simulink model "powers"  (Simulink 5.0)
settings: Solver=ode45  SolverMode=SingleTasking  StartTime=0.0  StopTime=0.2  RelTol=1e-4  AbsTol=1e-8
CloseFcn:
  | ;slview('closediagram',bdroot);
settings Model: LastModifiedBy=Blue Phoenix  LimitDataPoints=off  BlockReductionOpt=off  BooleanDataType=off

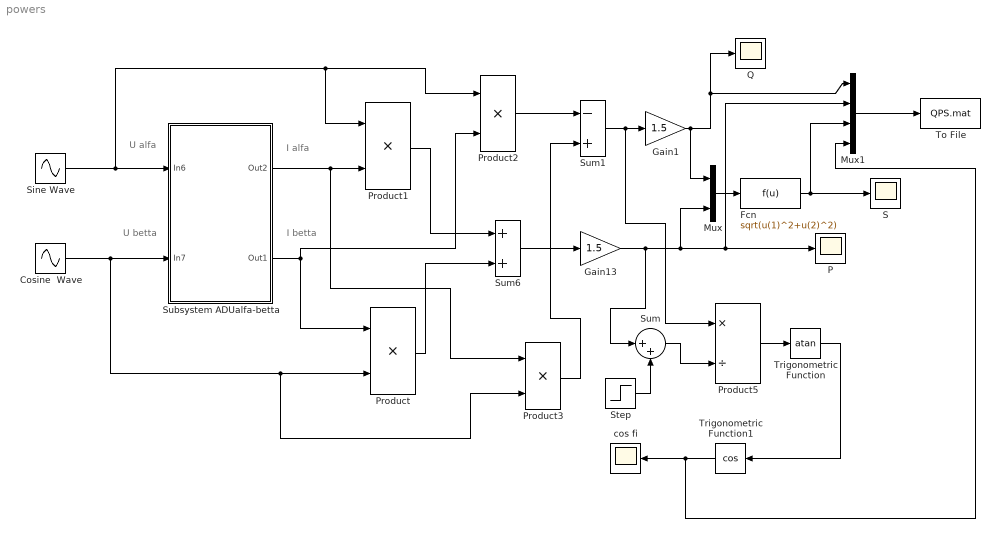
== system powers ==
  note: I alfa
  note: I betta
  note: U alfa
  note: U betta
  "  Q" : Scope
      settings: TickLabels=on  TimeRange=80  YMin=-1  YMax=2  SaveName=ScopeData3  DataFormat=Array
  "  S" : Scope
      settings: TickLabels=on  TimeRange=80  YMin=-1  YMax=2  SaveName=ScopeData5  DataFormat=Array
  " P" : Scope
      settings: TickLabels=on  TimeRange=80  YMin=-1  YMax=2  SaveName=ScopeData2  DataFormat=Array
  Cosine  Wave : Sin  Amplitude=311  Frequency=314  Phase=-pi/2  SampleTime=0
  Fcn : Fcn  Expr=sqrt(u(1)^2+u(2)^2)
  Gain1 : Gain  Gain=1.5  SaturateOnIntegerOverflow=on
  Gain13 : Gain  Gain=1.5  SaturateOnIntegerOverflow=on
  Mux : Mux  Inputs=2
  Mux1 : Mux
  Product{,1..3} (4 alike) : Product  SaturateOnIntegerOverflow=on  InputSameDT=on
  Product5 : Product  Inputs=*/  SaturateOnIntegerOverflow=on  InputSameDT=on
  Sine Wave : Sin  Amplitude=311  Frequency=314  SampleTime=0
  Step : Step  Time=0.001  Before=0.0001  After=0  SampleTime=0
  Subsystem ADUalfa-betta : Subsystem
  Sum : Sum  Inputs=|++  SaturateOnIntegerOverflow=on  InputSameDT=on
  Sum1 : Sum  Inputs=-+  SaturateOnIntegerOverflow=on  InputSameDT=on
  Sum6 : Sum  SaturateOnIntegerOverflow=on  InputSameDT=on
  To File : ToFile  Filename=QPS.mat
  Trigonometric Function : Trigonometry  Operator=atan
  Trigonometric Function1 : Trigonometry  Orientation=left  Operator=cos
  cos fi : Scope
      settings: TickLabels=on  TimeRange=0.1  YMin=-1  YMax=2  SaveName=ScopeData4  DataFormat=Array
  wires:
  Subsystem ADUalfa-betta/1(Out2) -> Product1/2, Product3/1
  Sine Wave/1 -> Subsystem ADUalfa-betta/1(In6), Product1/1, Product2/1
  Cosine  Wave/1 -> Subsystem ADUalfa-betta/2(In7), Product/2, Product3/2
  Subsystem ADUalfa-betta/2(Out1) -> Product/1, Product2/2
  Product1/1 -> Sum6/1
  Product/1 -> Sum6/2
  Gain13/1 -> Sum/1, Mux/2, " P"/1, Mux1/2
  Sum6/1 -> Gain13/1
  Product3/1 -> Sum1/2
  Product2/1 -> Sum1/1
  Sum1/1 -> Gain1/1, Product5/1
  Gain1/1 -> Mux/1, "  Q"/1, Mux1/1
  Product5/1 -> Trigonometric Function/1
  Trigonometric Function/1 -> Trigonometric Function1/1
  Step/1 -> Sum/2
  Sum/1 -> Product5/2
  Mux/1 -> Fcn/1
  Fcn/1 -> "  S"/1, Mux1/3
  Mux1/1 -> To File/1
  Trigonometric Function1/1 -> cos fi/1, Mux1/4

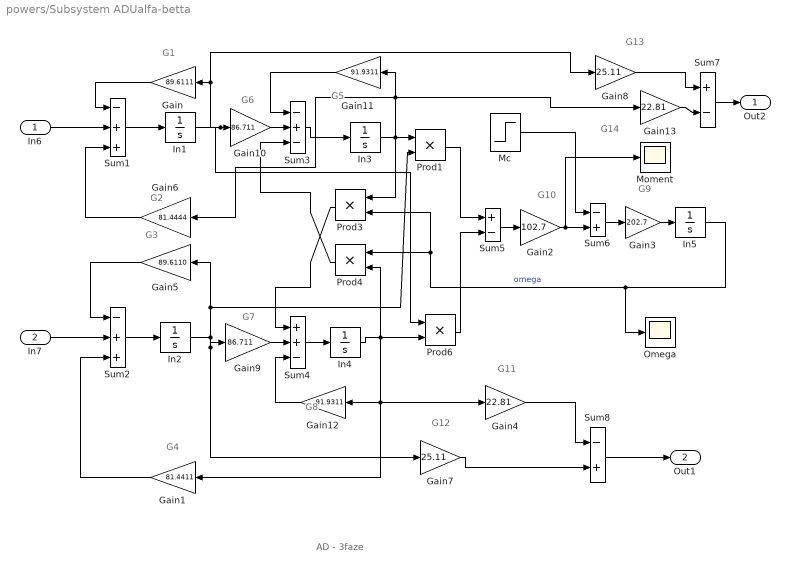
== system powers/Subsystem ADUalfa-betta ==
  note: G1
  note: G2
  note: G3
  note: G4
  note: G10
  note: G9
  note: G6
  note: G7
  note: G8
  note: G5
  note: AD - 3faze
  note: G14
  note: G12
  note: G13
  note: G11
  In6 : Inport
  In7 : Inport  Port=2
  "  Prod1" : Product  SaturateOnIntegerOverflow=on  InputSameDT=on
  Gain : Gain  Orientation=left  Gain=89.6111  SaturateOnIntegerOverflow=on
  Gain1 : Gain  Orientation=left  Gain=81.4411  SaturateOnIntegerOverflow=on
  Gain10 : Gain  Gain=86.711  SaturateOnIntegerOverflow=on
  Gain11 : Gain  Orientation=left  Gain=91.9311  SaturateOnIntegerOverflow=on
  Gain12 : Gain  Orientation=left  Gain=91.9311  SaturateOnIntegerOverflow=on
  Gain13 : Gain  Gain=22.81  SaturateOnIntegerOverflow=on
  Gain2 : Gain  Gain=102.7  SaturateOnIntegerOverflow=on
  Gain3 : Gain  Gain=202.7  SaturateOnIntegerOverflow=on
  Gain4 : Gain  Gain=22.81  SaturateOnIntegerOverflow=on
  Gain5 : Gain  Orientation=left  Gain=89.6110  SaturateOnIntegerOverflow=on
  Gain6 : Gain  Orientation=left  Gain=81.4444  SaturateOnIntegerOverflow=on
  Gain7 : Gain  Gain=25.11  SaturateOnIntegerOverflow=on
  Gain8 : Gain  Gain=25.11  SaturateOnIntegerOverflow=on
  Gain9 : Gain  Gain=86.711  SaturateOnIntegerOverflow=on
  In{1..5} (5 alike) : Integrator
  Mc : Step  Time=0.1  Before=0.0  After=10  SampleTime=0
  Moment : Scope
      settings: TickLabels=on  TimeRange=80  YMin=-1  YMax=2  DataFormat=Array
  Omega : Scope
      settings: TickLabels=on  TimeRange=0.2  YMin=-100  YMax=125  DataFormat=Array
  Prod3 : Product  Orientation=left  SaturateOnIntegerOverflow=on  InputSameDT=on
  Prod4 : Product  Orientation=left  SaturateOnIntegerOverflow=on  InputSameDT=on
  Prod6 : Product  SaturateOnIntegerOverflow=on  InputSameDT=on
  Sum1 : Sum  Inputs=-++  SaturateOnIntegerOverflow=on  InputSameDT=on
  Sum2 : Sum  Inputs=-++  SaturateOnIntegerOverflow=on  InputSameDT=on
  Sum3 : Sum  Inputs=-+-  SaturateOnIntegerOverflow=on  InputSameDT=on
  Sum4 : Sum  Inputs=++-  SaturateOnIntegerOverflow=on  InputSameDT=on
  Sum5 : Sum  Inputs=+-  SaturateOnIntegerOverflow=on  InputSameDT=on
  Sum6 : Sum  Inputs=-+  SaturateOnIntegerOverflow=on  InputSameDT=on
  Sum7 : Sum  Inputs=+-  SaturateOnIntegerOverflow=on  InputSameDT=on
  Sum8 : Sum  Inputs=-+  SaturateOnIntegerOverflow=on  InputSameDT=on
  Out2 : Outport
  Out1 : Outport  Port=2
  wires:
  Gain/1 -> Sum1/1
  Sum2/1 -> In2/1
  In4/1 -> Prod4/2, Prod6/2, Gain1/1, Gain12/1, Gain4/1
  In3/1 -> Prod3/1, "  Prod1"/1, Gain6/1, Gain11/1, Gain13/1
  Prod6/1 -> Sum5/2
  Sum6/1 -> Gain3/1
  Gain3/1 -> In5/1
  Mc/1 -> Sum6/1
  "  Prod1"/1 -> Sum5/1
  Sum3/1 -> In3/1
  Sum5/1 -> Gain2/1
  Sum1/1 -> In1/1
  In2/1 -> "  Prod1"/2, Gain5/1, Gain9/1, Gain7/1
  In1/1 -> Gain10/1, Gain/1, Gain8/1, Prod6/1
  Gain10/1 -> Sum3/2
  Gain9/1 -> Sum4/2
  Gain5/1 -> Sum2/1
  Prod4/1 -> Sum3/3
  Prod3/1 -> Sum4/1
  Gain2/1 -> Sum6/2, Moment/1
  Gain11/1 -> Sum3/1
  Gain12/1 -> Sum4/3
  In5/1 -> Prod3/2, Prod4/1, Omega/1  "omega"
  Sum4/1 -> In4/1
  Gain7/1 -> Sum8/2
  Gain4/1 -> Sum8/1
  Gain6/1 -> Sum1/3
  Gain1/1 -> Sum2/3
  In7/1 -> Sum2/2
  Gain8/1 -> Sum7/1
  Gain13/1 -> Sum7/2
  In6/1 -> Sum1/2
  Sum8/1 -> Out1/1
  Sum7/1 -> Out2/1
